simulink model "dc_motor"  (R2025a)
settings: Solver=VariableStepAuto  StartTime=0.0  StopTime=5  RelTol=1e-3
libraries: spsDCVoltageSourceLib x4, spsDCMachineLib x1, sps_lib x1
settings Model: Creator=Yunus Tosun  LastModifiedBy=Yunus Tosun

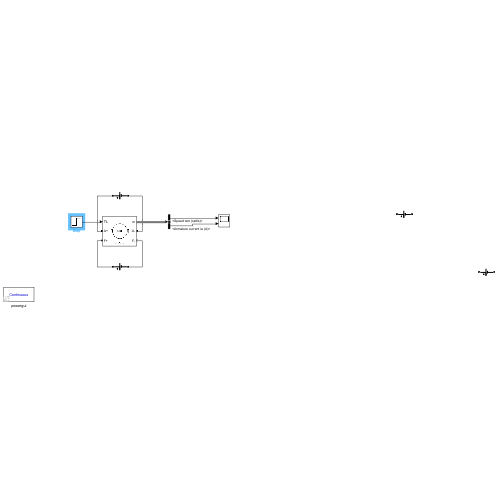
[thumbnail: Simulink's stored preview of the top-level diagram]
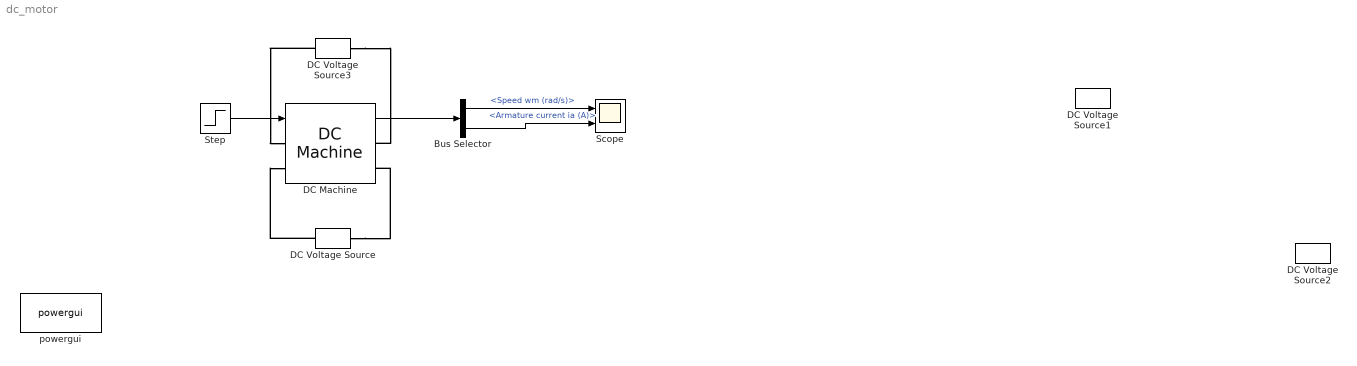
== system dc_motor ==
  Bus Selector : BusSelector  OutputSignals=Speed wm (rad/s),Armature current ia (A)
  DC Machine : spsDCMachineLib/DC Machine  PresetModel=No  MechanicalLoad=Torque TL  FieldType=Wound  ShowDetailedParameters=on  MeasurementBus=off  RLa="[ 1.07  0.0245]"  RLf="[ 210  23]"  Laf=1.18  MachineConstant=Torque constant (N.m/A)  Ke=1.8  Kt=1.8  J=0.06  Bm=0.0032  Tf=0.3  w0=0  Ifinit=1.04761904761905  TsPowergui=0  TsBlock=-1
  DC Voltage Source : spsDCVoltageSourceLib/DC Voltage Source  Amplitude=220  Measurements=None
  DC Voltage Source1 : spsDCVoltageSourceLib/DC Voltage Source  Amplitude=200  Measurements=None
  DC Voltage Source2 : spsDCVoltageSourceLib/DC Voltage Source  Amplitude=200  Measurements=None
  DC Voltage Source3 : spsDCVoltageSourceLib/DC Voltage Source  Amplitude=220  Measurements=None
  Scope : Scope  NumInputPorts=2
      settings: ActiveDisplayYMinimum=-24.107071119837119  ActiveDisplayYMaximum=246.2854194069219
  Step : Step  Time=2  After=26.1  SampleTime=0
  powergui : sps_lib/powergui  Priority=1  SimulationMode=Continuous  SampleTime=50e-6  frequency=60  Iterations=50  frequencyindice=0  Pbase=100e6  ErrMax=1e-4  UnitsV=kV  UnitsW=MW  buscounter=0  FunctionMessages=off  echomessages=off  EnableUseOfTLC=off  CurrentSourceSwitches=off  DisableSnubberDevices=off  DisableRonSwitches=off  DisableVfSwitches=off  DisplayEquations=off  AutomaticDiscreteSolvers=off  SolverType=Tustin/Backward Euler (TBE)  Interpol=off  ExternalGateDelay=off  methode=off  Ts=100  x0status=blocks  SPID=on  SwTol=0  HookPort=off  NonlinearTolerance=1e-4  nMaxIteration=100  ContinueOnMaxIteration=off  RestoreLinks=warning  ResistiveCurrentMeasurement=off  Frange=[0:2:500]  Ylog=off  Xlog=on  ShowGrid=off  save=off  variable=ZData  structure=0  ZoomFFT=off  StartTime=0.0  cycles=1  DisplayStyle=1  fundamental=60  FreqAxis=off  MaxFrequency=1000  frequencyindicesteady=1  RmsSteady=1  display=off
  wires:
  Step/1 -> DC Machine/1
  DC Machine/1 -> Bus Selector/1
  Bus Selector/1 -> Scope/1  "<Speed wm (rad/s)>"
  Bus Selector/2 -> Scope/2  "<Armature current ia (A)>"
  connections:
  DC Voltage Source/LConn1 -- DC Machine/RConn2
  DC Voltage Source/RConn1 -- DC Machine/LConn2
  DC Voltage Source3/RConn1 -- DC Machine/LConn1
  DC Voltage Source3/LConn1 -- DC Machine/RConn1
